simulink model "loadcell"  (R2024b)
settings: Solver=FixedStepAuto  StartTime=0.0  StopTime=50  FixedStep=0.1  RelTol=1e-3  EnableMultiTasking=on
libraries: stm32f4xxblockslib x3, simulink x1, dspstat3 x1
settings Model: STM32="{\"DigitalPortRead\":[{\"ID\":\"test:4\"},{\"ID\":\"hall:4\"},{\"ID\":\"loadcell:4\"}],\"AnalogInput\":[{\"ID\":\"test:47\"},{\"ID\":\"hall:47\"},{\"ID\":\"loadcell:47\"}],\"DigitalPortWrite\":[{\"ID\":\"test:64\"},{\"ID\":\"hall:64\"},{\"ID\":\"loadcell:64\"}]}"  Creator=FREED  LastModifiedBy=FREED
settings OptimizationCC: DefaultParameterBehavior=Inlined  EnhancedBackFolding=on  PassReuseOutputArgsAs=Individual arguments  ZeroExternalMemoryAtStartup=off  ZeroInternalMemoryAtStartup=off  MaxStackSize=512  OptimizeBlockOrder=speed  DifferentSizesBufferReuse=on  OptimizationCustomize=off  EfficientTunableParamExpr=on
settings DebuggingCC: ParameterTunabilityLossMsg=error
settings HardwareCC: ProdBitPerPointer=32  ProdBitPerSizeT=32  ProdBitPerPtrDiffT=32  ProdLargestAtomicInteger=Long  ProdLargestAtomicFloat=Double  ProdWordSize=32  ProdLongLongMode=on  ProdHWDeviceType=ARM Compatible->ARM Cortex-M
settings SFSimCC: MATLABDynamicMemAlloc=off
settings RTWCC: Description=Embedded Coder  SystemTargetFile=ert.tlc  HardwareBoard=STM32G4xx Based  TemplateMakefile=ert_default_tmf  Toolchain=GNU Tools for ARM Embedded Processors
settings CodeAppCC: ForceParamTrailComments=on  IgnoreCustomStorageClasses=off  OperatorAnnotations=on  SimulinkDataObjDesc=on  SFDataObjDesc=on  InsertBlockDesc=on
settings ERTTargetCC: TargetLangStandard=C99 (ISO)  CodeReplacementLibrary=ARM Cortex-M  ExtModeTransport=3  ExtModeStaticAlloc=on  ExtModeStaticAllocSize=2048  ExtModeMexFile=ext_xcp  ExtModeIntrfLevel=Level2 - Open

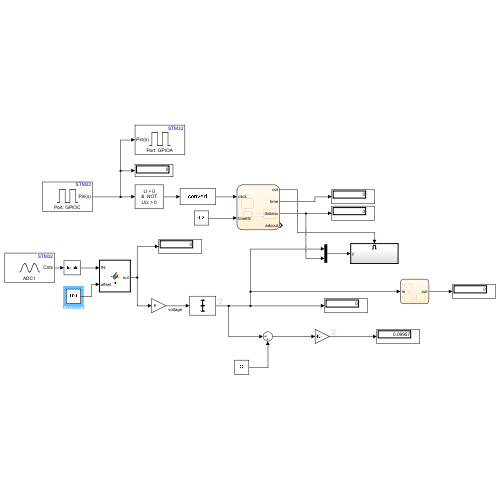
[thumbnail: Simulink's stored preview of the top-level diagram]
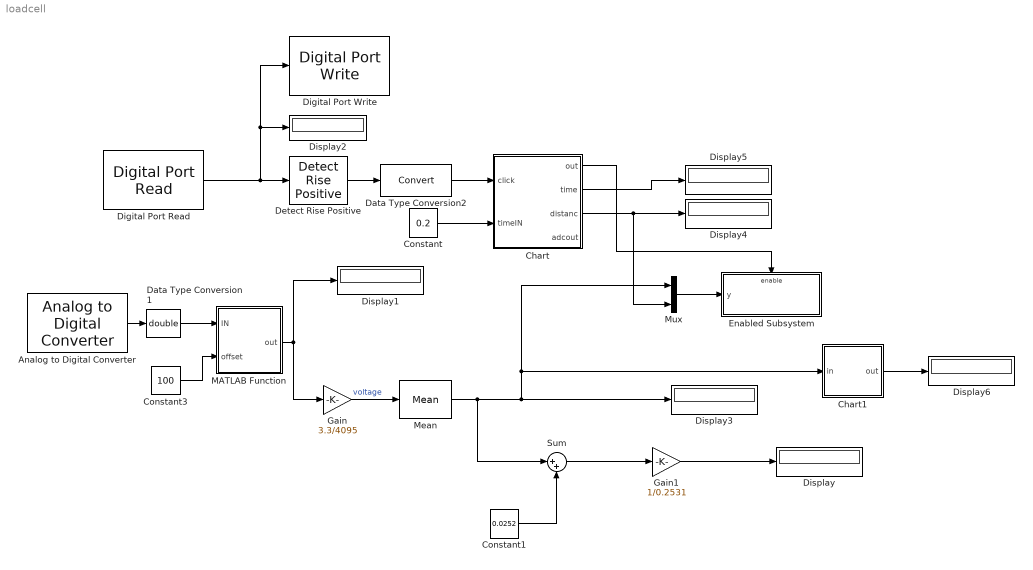
== system loadcell ==
  Analog to Digital Converter : stm32f4xxblockslib/Analog to Digital Converter  ADCModule=ADC1  ConversionGroup=Regular  TriggerMode=Trigger and read  NumberOfConversions=1  EnableBufferConv=off  BufferLength=1  OutputStatus=off  SampleTime=-1  EnableSimPort=off  hoistedMaskSrc=ECSoC/ECSimCodegen/Analog to Digital Converter
  Chart : Stateflow chart  TreatAsAtomicUnit=on
  Chart1 : Stateflow chart  TreatAsAtomicUnit=on
  Constant : Constant  Value=0.2
  Constant1 : Constant  Value=0.0252
  Constant3 : Constant  Value=100
  Data Type Conversion1 : DataTypeConversion  OutDataTypeStr=double  SaturateOnIntegerOverflow=off  RndMeth=Floor
  Data Type Conversion2 : DataTypeConversion  SaturateOnIntegerOverflow=off  RndMeth=Floor
  Detect Rise Positive : simulink/Logic and Bit Operations/Detect Rise Positive  vinit=0  OutDataTypeStr=boolean
  Digital Port Read : stm32f4xxblockslib/Digital Port Read  PortName=GPIOC  PinNumber=[13]  ReadOperation=on  IOAsArray=on  SampleTime=-1  EnableSimPort=off  hoistedMaskSrc=ECSoC/ECSimCodegen/Digital Port Read
      settings: LibrarySourceBlock=stm32g4xxblockslib/Digital Port Read
  Digital Port Write : stm32f4xxblockslib/Digital Port Write  PortName=GPIOA  PinNumber=[5]  ReadOperation=off  IOAsArray=on  EnableSimPort=off  hoistedMaskSrc=ECSoC/ECSimCodegen/Digital Port Write
      settings: LibrarySourceBlock=stm32g4xxblockslib/Digital Port Write
  Display{,1..6} (7 alike) : Display
  Enabled Subsystem : Subsystem  TreatAsAtomicUnit=on
  Gain : Gain  Gain=3.3/4095
  Gain1 : Gain  Gain=1/0.2531
  MATLAB Function : MATLAB Function  TreatAsAtomicUnit=on
  Mean : dspstat3/Mean  run=off  InputProcessing=Columns as channels (frame based)  reset_popup=None  directionMode=Each column  dimension=1  roiEnable=off  roiType=Rectangles  roiPortion=Entire ROI  roiOutput=Individual statistics for each ROI  roiFlag=off  roundingMode=Floor  overflowMode=off  outputDataTypeStr=Inherit: Same as accumulator  outputMin=[]  outputMax=[]  outputLastDataTypeStr=Inherit: Same as accumulator
  Mux : Mux  Inputs=2
  Sum : Sum  Inputs=|++
  wires:
  Digital Port Read/1 -> Digital Port Write/1, Display2/1, Detect Rise Positive/1
  Mean/1 -> Sum/1, Mux/1, Chart1/1(in), Display3/1
  Gain/1 -> Mean/1  "voltage"
  Chart/3(distanc) -> Mux/2, Display4/1
  Constant/1 -> Chart/2(timeIN)
  Chart/2(time) -> Display5/1
  Detect Rise Positive/1 -> Data Type Conversion2/1
  Chart/1(out) -> Enabled Subsystem/Enable
  Data Type Conversion2/1 -> Chart/1(click)
  Chart1/1(out) -> Display6/1
  MATLAB Function/1(out) -> Gain/1, Display1/1
  Constant3/1 -> MATLAB Function/2(offset)
  Analog to Digital Converter/1 -> Data Type Conversion1/1
  Data Type Conversion1/1 -> MATLAB Function/1(IN)
  Mux/1 -> Enabled Subsystem/1(y)
  Constant1/1 -> Sum/2
  Sum/1 -> Gain1/1
  Gain1/1 -> Display/1

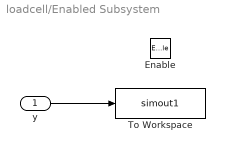
== system loadcell/Enabled Subsystem ==
  y : Inport
  Enable : EnablePort
  To Workspace : ToWorkspace  VariableName=simout1  SampleTime=-1
      settings: Save2DSignal=2-D array (concatenate along first dimension)
  wires:
  y/1 -> To Workspace/1

== stateflow chart loadcell/Chart1 ==
  state start
    out=0;
  state low
    entry:
    out=0
  state high
    entry:
    out=3.3
  (default) -> start
  start -> low : [in<=1]
  low -> high : [in > 2]
  high -> low : [in<1]
  data: out output; in input

== matlab function loadcell/MATLAB Function ==
  data: IN input; out output; offset input
function out  = fcn(IN,offset)

if (IN - offset) <0
    out = 0;
else
    out = IN - offset;
end

== stateflow chart loadcell/Chart ==
  state setup
    entry:
    time=0;
    out=0;
    distanc=0;
    adcout=0;
  state setup1
    entry:
    out=1;
    during:
    time=time+0.001;
    exit:
    distanc=distanc+500
  state start
    entry:
    time=0;
    out=0;
  (default) -> setup
  setup -> start
  setup1 -> start : [time>timeIN]
  start -> setup1 : [click == 1]
  data: click input; out output; time output; distanc output; timeIN input; adcout output
